simulink model "power_machines"  (Simulink 6.0)
settings: Solver=ode23tb  SolverMode=SingleTasking  StartTime=0.0  StopTime=5  RelTol=1e-3
undefined symbols (not defined in the file or in its folder): D1, Delta
libraries: powerlib x12
settings Model: Creator=patrice  LastModifiedBy=batserve  ExtModeTrigMode=oneshot  ExtModeArmWhenConnect=off  ExtModeAutoUpdateStatusClock=off  ProdHWDeviceType=Specified
settings DataIOCC: LimitDataPoints=off  SignalLoggingName=sigsOut  OutputTimes=[0:1/20:10]
settings OptimizationCC: BlockReduction=off  BooleanDataType=off  InlineInvariantSignals=off
settings DebuggingCC: CheckExecutionContextPreStartOutputMsg=on  CheckExecutionContextRuntimeOutputMsg=on  SolverPrmCheckMsg=none  UnconnectedLineMsg=none
settings HardwareCC: ProdBitPerShort=32  ProdBitPerInt=16  ProdHWDeviceType=Specified  TargetUnknown=on
settings RTWCC: TemplateMakefile=grt_unix.tmf
settings CodeAppCC: IgnoreCustomStorageClasses=off

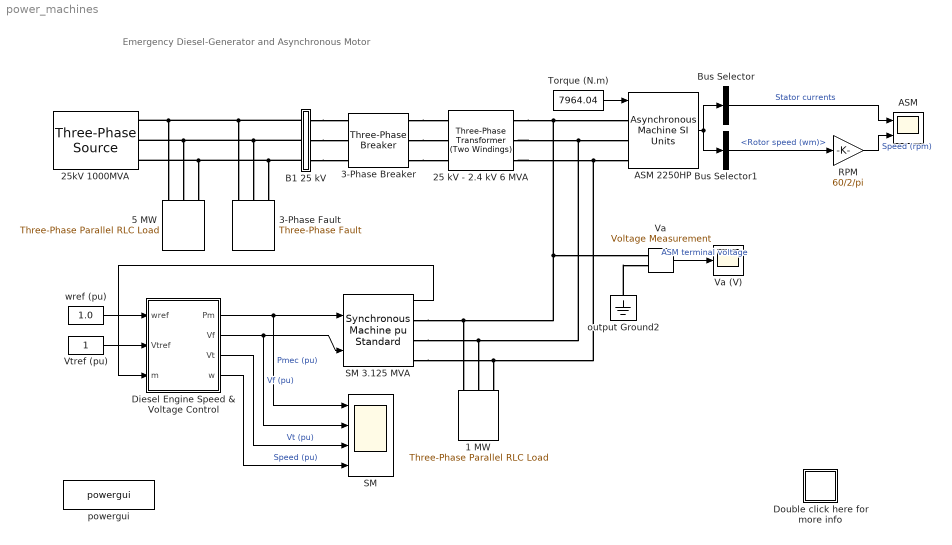
== system power_machines ==
  note: Emergency Diesel-Generator and Asynchronous Motor
  1 MW : powerlib/Elements/Three-Phase Parallel RLC Load  Orientation=down  PhysicalDomain=powersysdomain  SubClassName=unknown  LeftPortType=p1  RightPortType=p1  LConnTagsString=A|B|C  Configuration=Y (grounded)  NominalVoltage=2400  NominalFrequency=60  ActivePower=1e6  InductivePower=0  CapacitivePower=0  Measurements=None
  25 kV - 2.4 kV 6 MVA : powerlib/Elements/Three-Phase Transformer (Two Windings)  NominalPower=[ 6e6 , 60 ]  Winding1Connection=Yg  Winding1=[ 25e3 , 0.0015 , 0.03]  Winding2Connection=Delta (D1)  Winding2=[ 2.4e3 , 0.0015 , 0.03 ]  SetSaturation=off  Rm=200  Lm=200  Saturation="[ 0,0  ;  0.005,1.2  ;  1.0,1.4 ]"  Hysteresis=off  DataFile='hysteresis'  SetInitialFlux=off  InitialFluxes=[ 0.8 , -0.8 , 0.7 ]  Measurements=None  TransfoNumber=0
  25kV 1000MVA : powerlib/Electrical Sources/Three-Phase Source  Voltage=25e3  PhaseAngle=0  Frequency=60  InternalConnection=Yg  SpecifyImpedance=on  Resistance=25^2/1000/10  Inductance=25^2/1000/377  ShortCircuitLevel=1000e6  BaseVoltage=25e3  XRratio=10
  3-Phase Breaker : powerlib/Elements/Three-Phase Breaker  InitialState=closed  SwitchA=on  SwitchB=on  SwitchC=on  SwitchTimes=[0.2]  External=off  BreakerResistance=0.01  SnubberResistance=1e5  SnubberCapacitance=inf  Measurements=None
      settings: AttributesFormatString=\n
  3-Phase Fault : powerlib/Elements/Three-Phase Fault  Orientation=down  FaultA=on  FaultB=on  FaultC=on  FaultResistance=0.01  GroundFault=on  GroundResistance=0.001  External=off  SwitchStatus=[1 0]  SwitchTimes=[ 0.1 0.4]  InitialStates=[1 1 0]  SnubberResistance=inf  SnubberCapacitance=inf  Measurements=None
  5 MW : powerlib/Elements/Three-Phase Parallel RLC Load  Orientation=down  PhysicalDomain=powersysdomain  SubClassName=unknown  LeftPortType=p1  RightPortType=p1  LConnTagsString=A|B|C  Configuration=Y (grounded)  NominalVoltage=25e3  NominalFrequency=60  ActivePower=5e6  InductivePower=0  CapacitivePower=0  Measurements=None
  ASM : Scope  NumInputPorts=2
      settings: TimeRange=0.2  YMin=-5000~-70  YMax=6000~0  DataFormat=Array
  ASM 2250HP : powerlib/Machines/Asynchronous Machine SI Units  PresetModel=No  ShowDetailedParameters=on  RotorType=Squirrel-cage  ReferenceFrame=Rotor  NominalParameters=[ 2250*746, 2400, 60 ]  Stator=[ 0.029 0.226/377]  Rotor=[ 0.022 0.226/377]  Lm=13.04/377  Mechanical="[ 63.87 0  2 ]"  InitialConditions=[1 0 0 0 0 0 0 0]  Units=1  LoadFlowParameters=1492000
  B1 25 kV : Subsystem
      mask Display: disp('')
  Bus Selector : BusSelector  DialogController=Simulink.DDGSource_Bus  OutputSignals=Stator measurements.Stator current is_a (A),Stator measurements.Stator current is_b (A),Stator measurements.Stator current is_c (A)  MuxedOutput=on
  Bus Selector1 : BusSelector  DialogController=Simulink.DDGSource_Bus  OutputSignals=Mechanical.Rotor speed (wm)
  Diesel Engine Speed & Voltage Control : Subsystem
  Double click here for more info : Subsystem
      mask Display: disp('?')
  RPM : Gain  Gain=60/2/pi  SaturateOnIntegerOverflow=on
  SM : Scope  NumInputPorts=4
      settings: TimeRange=0.8  YMin=0~0~0~0.8  YMax=1.5~6~1.5~1.2  SaveName=Pmec_SM  DataFormat=Structure  Decimation=10
  SM 3.125 MVA : powerlib/Machines/Synchronous Machine pu Standard  PresetModel=No  ShowDetailedParameters=on  RotorType=Salient-pole  NominalParameters="[ 3.125e6  2400  60]"  Reactances1=[ 31 32 33 34 35 36 37 ]  Reactances2=[ 1.56, 0.296, 0.177, 1.06, 0.177, 0.052 ]  dAxisTimeConstants=Short-circuit  qAxisTimeConstants=Open-circuit  TimeConstants1=[]  TimeConstants2=[]  TimeConstants3=[]  TimeConstants4=[]  TimeConstants5=[ 3.7, 0.05, 0.05 ]  TimeConstants6=[]  TimeConstants7=[0.024 0.006 0.006]  TimeConstants8=[]  StatorResistance=0.0036  Mechanical="[ 1.07  0  2 ]"  InitialConditions=[0 0 0 0 0 0 0 0 1]  SetSaturation=off  Saturation=[0.211 0.418 1.0 1.72 3.35 ; 0.25 0.50 1.0 1.2 1.4]  Units=0.5  LoadFlowParameters=[1 0 0 0]
      settings: AttributesFormatString=\n\n
  Torque (N.m) : Constant  Value=7964.04
  Va : powerlib/Measurements/Voltage Measurement  Tag=PoWeRsYsTeMmEaSuReMeNt  PhasorSimulation=off  OutputType=Magnitude  PSBequivalent=0
  Va (V) : Scope
      settings: TickLabels=on  TimeRange=0.2  YMin=-2000  YMax=2000  DataFormat=Array
  Vtref (pu) : Constant
  output Ground2 : powerlib/Elements/Ground  Orientation=down  PhysicalDomain=powersysdomain  SubClassName=unknown  LeftPortType=p1  RightPortType=p1  LConnTagsString=a
  powergui : powerlib/powergui  Priority=2  Frange=logspace(0,3,50)  Ylog=off  Xlog=off  save=off  variable=ZData  ZoomFFT=on  StartTime=0.0  cycles=2  DisplayStyle=off  fundamental=60  FreqAxis=off  MaxFrequency=1000  frequencyindice=60  frequencyindicesteady=1  RmsSteady=1  display=off  Ts=0  methode=off  frequency=60  echomessages=on
  wref (pu) : Constant  Value=1.0
  wires:
  wref (pu)/1 -> Diesel Engine Speed & Voltage Control/1(wref)
  Vtref (pu)/1 -> Diesel Engine Speed & Voltage Control/2(Vtref)
  Diesel Engine Speed & Voltage Control/3(Vt) -> SM/3  "Vt (pu)"
  Diesel Engine Speed & Voltage Control/4(w) -> SM/4  "Speed (pu)"
  SM 3.125 MVA/1 -> Diesel Engine Speed & Voltage Control/3(m)
  Torque (N.m)/1 -> ASM 2250HP/1
  ASM 2250HP/1 -> Bus Selector/1, Bus Selector1/1
  Va/1 -> Va (V)/1  "ASM terminal voltage"
  Diesel Engine Speed & Voltage Control/1(Pm) -> SM 3.125 MVA/1, SM/1  "Pmec (pu)"
  Diesel Engine Speed & Voltage Control/2(Vf) -> SM 3.125 MVA/2, SM/2  "Vf (pu)"
  Bus Selector/1 -> ASM/1  "Stator currents"
  Bus Selector1/1 -> RPM/1  "<Rotor speed (wm)>"
  RPM/1 -> ASM/2  "Speed (rpm)"
  connections:
  B1 25 kV/LConn3 -- 3-Phase Fault/LConn3 -- 25kV 1000MVA/RConn3 -- 5 MW/LConn3
  B1 25 kV/LConn2 -- 3-Phase Fault/LConn2 -- 25kV 1000MVA/RConn2 -- 5 MW/LConn2
  B1 25 kV/LConn1 -- 3-Phase Fault/LConn1 -- 25kV 1000MVA/RConn1 -- 5 MW/LConn1
  B1 25 kV/RConn3 -- 3-Phase Breaker/LConn3
  B1 25 kV/RConn2 -- 3-Phase Breaker/LConn2
  B1 25 kV/RConn1 -- 3-Phase Breaker/LConn1
  3-Phase Breaker/RConn1 -- 25 kV - 2.4 kV 6 MVA/LConn1
  3-Phase Breaker/RConn3 -- 25 kV - 2.4 kV 6 MVA/LConn3
  3-Phase Breaker/RConn2 -- 25 kV - 2.4 kV 6 MVA/LConn2
  output Ground2/LConn1 -- Va/LConn2
  SM 3.125 MVA/RConn2 -- 25 kV - 2.4 kV 6 MVA/RConn2 -- ASM 2250HP/LConn2 -- 1 MW/LConn2
  SM 3.125 MVA/RConn1 -- 1 MW/LConn1 -- 25 kV - 2.4 kV 6 MVA/RConn1 -- ASM 2250HP/LConn1 -- Va/LConn1
  SM 3.125 MVA/RConn3 -- 25 kV - 2.4 kV 6 MVA/RConn3 -- ASM 2250HP/LConn3 -- 1 MW/LConn3

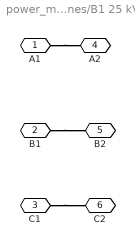
== system power_machines/B1 25 kV ==
  A1 : PMIOPort  Port=1  Side=Left
  B1 : PMIOPort  Port=2  Side=Left
  C1 : PMIOPort  Port=3  Side=Left
  A2 : PMIOPort  Orientation=left  Port=4  Side=Right
  B2 : PMIOPort  Orientation=left  Port=5  Side=Right
  C2 : PMIOPort  Orientation=left  Port=6  Side=Right
  connections:
  C1/RConn1 -- C2/RConn1
  B1/RConn1 -- B2/RConn1
  A1/RConn1 -- A2/RConn1

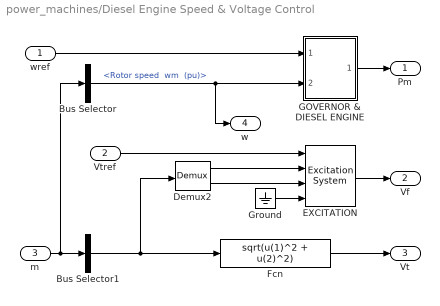
== system power_machines/Diesel Engine Speed & Voltage Control ==
  wref : Inport  Port=1  LatchInput=off
  Vtref : Inport  Port=2  LatchInput=off
  m : Inport  Port=3  LatchInput=off
  Bus Selector : BusSelector  DialogController=Simulink.DDGSource_Bus  OutputSignals="Mechanical.Rotor speed  wm  (pu)"
  Bus Selector1 : BusSelector  DialogController=Simulink.DDGSource_Bus  OutputSignals="dq0 components.Stator voltage  vd (pu),dq0 components.Stator voltage  vq (pu)"  MuxedOutput=on
  Demux2 : Demux  Outputs=2
  EXCITATION : powerlib/Machines/Excitation System  tr=20e-3  reg=[ 200, 0.02 ]  exc=[ 1, 0 ]  tgr=[ 0, 0 ]  damp=[ 0.001, 0.1 ]  sat=[ 0, 0 ]  lim=[ 0, 6, 0 ]  v0=[1,1.42734]
  Fcn : Fcn  Expr=sqrt(u(1)^2 + u(2)^2)
  GOVERNOR & DIESEL ENGINE : Subsystem  mask(Diesel Engine & Governor){K=40, Tr=[0.01 0.02 0.2], Ta=[0.25 0.009 0.0384], Tlim=[0 1.1], Td=0.024, Pm0=0.000270147}
      mask prompts: K "Regulator gain K:"; Tr "Regulator time constants [T1 T2 T3 ] (s) :"; Ta "Actuator time constants [T4 T5 T6] (s) :"; Tlim "Torque limits [Tmin Tmax] (pu) :"; Td "Engine time delay Td (s) :"; Pm0 "Initial value of mechanical power  Pm0 (pu) :"
      mask help:
      | This block implements a diesel engine and governor system:
      | 1st and 2nd inputs: Desired and actual speed (pu)
      | Output: Diesel engine mechanical power.Motor inertia should be combined with generator.
      | Controller transfer function:
      |      Hc=K.(1+T3.s)/(1+T1.s+T1.T2.s^2)
      | Actuator transfer function :
      |      Ha= (1+T4.s) / [ (s (1+T5.s)(1+T6.s) ]
      | Motor :
      |      Time delay Td
      |
      | (See reference in Tutorial Session 5)
  Ground : Ground
  Pm : Outport  InitialOutput=0
  Vf : Outport  Port=2  InitialOutput=0
  Vt : Outport  Port=3  InitialOutput=0
  w : Outport  Port=4  InitialOutput=0
  wires:
  Ground/1 -> EXCITATION/4
  m/1 -> Bus Selector/1, Bus Selector1/1
  wref/1 -> GOVERNOR & DIESEL ENGINE/1(wref (pu))
  Demux2/2 -> EXCITATION/3
  EXCITATION/1 -> Vf/1
  GOVERNOR & DIESEL ENGINE/1(Pmec (pu)) -> Pm/1
  Vtref/1 -> EXCITATION/1
  Demux2/1 -> EXCITATION/2
  Bus Selector1/1 -> Demux2/1, Fcn/1
  Fcn/1 -> Vt/1
  Bus Selector/1 -> GOVERNOR & DIESEL ENGINE/2(w (pu)), w/1  "<Rotor speed  wm  (pu)>"

== system power_machines/Double click here for more info ==
  note: Open the SM and ASM scopes displaying the synchronous machine and asynchronous machine signals.  Start the simulation.
      | Observe that during the fault the terminal voltage drops to about 0.2 pu and the excitation voltage hits the limit of 6 pu. After fault clearing and islanding
      | the SM  mechanical power  increases from its initial value of  0 pu to the final value of 0.80 pu required by the resistive and motor load (2.49 MW). After 3 seconds,
      | the terminal voltage stabilizes at 1 pu. The motor speed decreases transiently from 1789 rpm to 1635 rpm, then it recovers close to its normal value after 2 seconds.
      |
      | If you  increase the fault duration to 12 cycles by changing the breaker opening time to 0.3 s, you will notice that the system collapses.
      | The ASM speed slows down to zero after 2 seconds.
  note: 3
  note: 1
  note: Demonstration
  note: Circuit Description
  note: This demonstration illustrates fault and islanding of an induction motor/diesel-generator system
      | and demonstrates the Machine Load Flow option of the Powergui.  (See Chapter 2 of the User's Guide.)
  note: A plant consisting of a resistive and motor load (ASM) is fed at 2400 V from a distibution 25 kV network through a 6 MVA 25/2 kV Wye-Delta transformer and from an
      | emergency synchronous generator/ diesel engine unit (SM). The 25 kV network is modelled by a simple R-L equivalent source (short-circuit level 1000 MVA) and a 5 MW load.
      | The  asynchronous motor is  rated 2250 HP, 2.4 kV and the synchronous machine is rated 3.125 MVA, 2.4kV. The SM excitation is performed by the standard
      | excitation block provided in the machine library. The diesel engine and governor system are modelled by a Simulink block (See tutorial, session 7 in the User`s Guide).
      | Initially, the motor develops a mechanical power of 2000 HP (1.49 MW) and the diesel generator is in standby, providing no active power.The synchronous machine excitation
      | system controls the 2400 V bus B2 voltage at 1 pu.  At t = 0.1 s, a three-phase to ground fault occurs on the 25 kV system, causing opening of the 25kV circuit breaker at t = 0.2 s.
      |
      | The demonstration illustrates the mechanical and electrical transients following the fault and islanding of the Motor/Generator system.
  note: Start Simulation. If the SM and ASM initial conditions are not properly set, you observe that the voltage and currents Machine do not start in steady state.
      | Stop the simulation.
  note: 2
  note: In order to start the simulation in steady-state, you must initialize the synchronous machine and the asynchronous motor for the desired load flow.
      | Open the  Powergui and select "Load Flow & Machine initialization" . The machine "Bus type" should be already initialized as "PV generator",
      | indicating that  the load flow will be performed with the machine controlling its active power and terminal voltage. Specify the desired values by entering
      | the following parameters:
  note: The diesel engine governor and SM excitation system contain integrators and transfer functions which have also been initialized  by the load flow.
      | Open the GOVERNOR block in the Diesel Engine subsystem. Note that the initial mechanical power has been automatically set to 0.00027 pu (844 W).
      | Now open the EXCITATION block. Notice in the last line of the block menu, that the initial terminal voltage Vt0 and field voltage Vf0  have been set respectively to
      | 1.0 and 1.4273 pu.The value of the constant block connnected to the torque input of the asynchronous motor has also been automatically set to 7964 N.
  note: 4
  note: G. Sybille (Hydro-Quebec)
  note: Load Flow : U AB (Vrms) = 2400 , P (wattts) = 0. Specify also the ASM mechanical power by entering Pmec (Watts) = 2000*746.
  note: Then press the "Execute Load Flow" button.
      |
      | Once the load flow is solved, the three line-to-line machine voltages and the three machine currents are updated.
      | The SM reactive power,  mechanical power and  field voltage are displayed: Q = 856 kvar; Pmec = 844 W (power required by resistive losses in stator winding );
      |  field voltage Ef = 1.4273 pu; the active and reactive powers absorbed by the motor, slip and torque are also displayed.

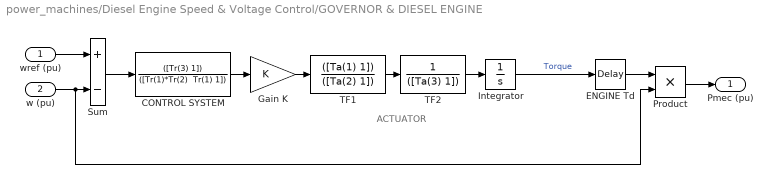
== system power_machines/Diesel Engine Speed & Voltage Control/GOVERNOR & DIESEL ENGINE ==
  note: ACTUATOR
  wref (pu) : Inport  Port=1  LatchInput=off
  w (pu) : Inport  Port=2  LatchInput=off
  CONTROL SYSTEM : TransferFcn  Numerator=([Tr(3) 1])  Denominator="([Tr(1)*Tr(2)  Tr(1) 1])"
  ENGINE Td : TransportDelay  DelayTime=Td  InitialInput=Pm0
  Gain K : Gain  Gain=K  SaturateOnIntegerOverflow=on
  Integrator : Integrator  InitialCondition=Pm0  LimitOutput=on  UpperSaturationLimit=Tlim(2)  LowerSaturationLimit=Tlim(1)
  Product : Product  SaturateOnIntegerOverflow=on  InputSameDT=on
  Sum : Sum  Inputs=+-  SaturateOnIntegerOverflow=on  InputSameDT=on
  TF1 : TransferFcn  Numerator=([Ta(1) 1])  Denominator=([Ta(2) 1])
  TF2 : TransferFcn  Numerator=1  Denominator=([Ta(3) 1])
  Pmec (pu) : Outport  InitialOutput=0
  wires:
  Gain K/1 -> TF1/1
  Sum/1 -> CONTROL SYSTEM/1
  CONTROL SYSTEM/1 -> Gain K/1
  TF1/1 -> TF2/1
  w (pu)/1 -> Product/2, Sum/2
  ENGINE Td/1 -> Product/1
  wref (pu)/1 -> Sum/1
  Product/1 -> Pmec (pu)/1
  TF2/1 -> Integrator/1
  Integrator/1 -> ENGINE Td/1  "Torque"
